simulink subsystem "Motor_drive_1D"  (R2024a)
settings: Solver=VariableStepAuto  StartTime=0.0  StopTime=10.0  RelTol=1e-3
undefined symbols (not defined in the file or in its folder): D_min
settings Model: Creator=Peter  LastModifiedBy=Peter

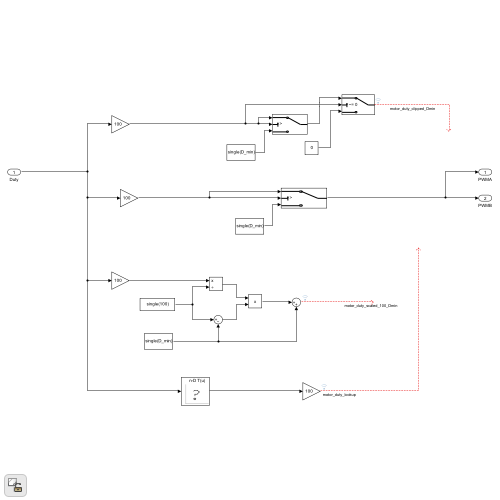
[thumbnail: Simulink's stored preview of the top-level diagram]
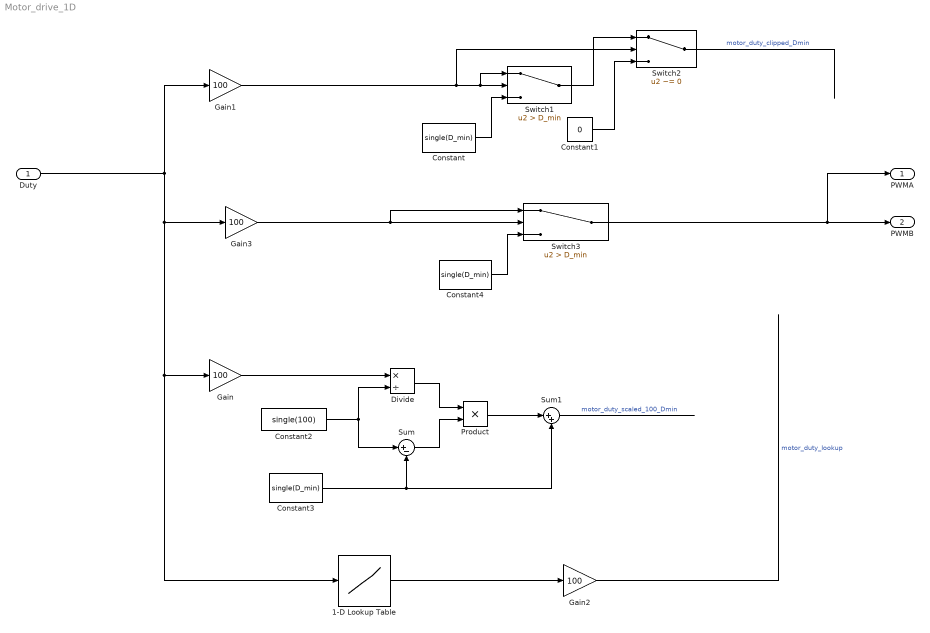
== system Motor_drive_1D ==
  Duty : Inport  OutDataTypeStr=single
  1-D Lookup Table : Lookup_n-D  NumberOfTableDimensions=1  BreakpointsForDimension1=[0:0.01:1]  Table=D_min/100*tanh([0:0.01:1]/0.05)+(100-D_min)/100*[0:0.01:1]  InternalRulePriority=Speed  RndMeth=Simplest
  Constant : Constant  Value=single(D_min)  OutDataTypeStr=single
  Constant1 : Constant  Value=0  OutDataTypeStr=single
  Constant2 : Constant  Value=single(100)  OutDataTypeStr=single
  Constant3 : Constant  Value=single(D_min)  OutDataTypeStr=single
  Constant4 : Constant  Value=single(D_min)  OutDataTypeStr=single
  Divide : Product  Inputs=*/
  Gain{,1..3} (4 alike) : Gain  Gain=100
  Product : Product
  Sum : Sum  Inputs=|+-
  Sum1 : Sum  Inputs=|++
  Switch1 : Switch  Criteria=u2 > Threshold  Threshold=D_min  OutDataTypeStr=single  SaturateOnIntegerOverflow=off  InputSameDT=off
  Switch2 : Switch  Criteria=u2 ~= 0  OutDataTypeStr=single  SaturateOnIntegerOverflow=off  InputSameDT=off
  Switch3 : Switch  Criteria=u2 > Threshold  Threshold=D_min  OutDataTypeStr=single  SaturateOnIntegerOverflow=off  InputSameDT=off
  PWMA : Outport  OutDataTypeStr=single
  PWMB : Outport  Port=2  OutDataTypeStr=single
  wires:
  Duty/1 -> Gain/1, 1-D Lookup Table/1, Gain3/1, Gain1/1
  Constant/1 -> Switch1/3
  Switch1/1 -> Switch2/1
  Constant1/1 -> Switch2/3
  Constant2/1 -> Divide/2, Sum/1
  Constant3/1 -> Sum/2, Sum1/2
  Sum/1 -> Product/2
  Divide/1 -> Product/1
  Product/1 -> Sum1/1
  Sum1/1 -> ?  "motor_duty_scaled_100_Dmin"
  Switch2/1 -> ?  "motor_duty_clipped_Dmin"
  1-D Lookup Table/1 -> Gain2/1
  Gain/1 -> Divide/1
  Gain1/1 -> Switch1/1, Switch1/2, Switch2/2
  Gain2/1 -> ?  "motor_duty_lookup"
  Gain3/1 -> Switch3/1, Switch3/2
  Constant4/1 -> Switch3/3
  Switch3/1 -> PWMB/1, PWMA/1
